simulink model "counter_block"  (R2016b)
settings: Solver=VariableStepAuto  StartTime=0.0  StopTime=10.0  RelTol=1e-3
settings Model: Creator=Lupus  LastModifiedBy=Lupus

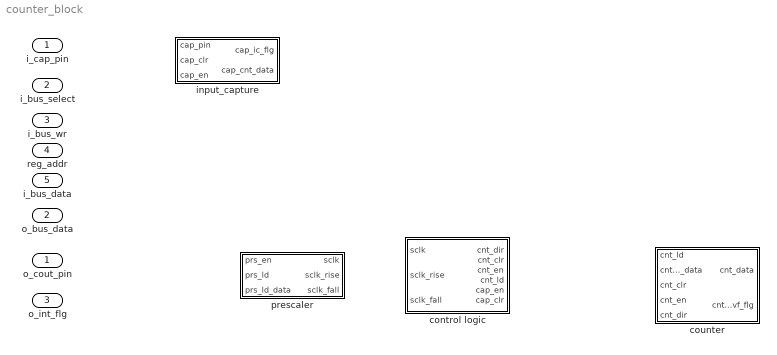
== system counter_block ==
  i_cap_pin : Inport
  i_bus_select : Inport  Port=2
  i_bus_wr : Inport  Port=3
  reg_addr : Inport  Port=4
  i_bus_data : Inport  Port=5
  "control logic " : Subsystem
  counter : Subsystem
  input_capture : Subsystem
  prescaler : Subsystem
  o_cout_pin : Outport
  o_bus_data : Outport  Port=2
  o_int_flg : Outport  Port=3

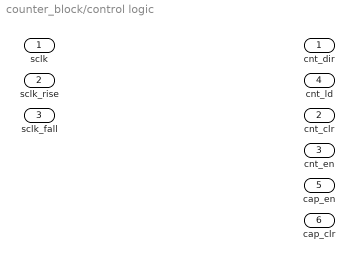
== system counter_block/control logic  ==
  sclk : Inport
  sclk_rise : Inport  Port=2
  sclk_fall : Inport  Port=3
  cnt_dir : Outport
  cnt_clr : Outport  Port=2
  "cnt_en " : Outport  Port=3
  cnt_ld : Outport  Port=4
  cap_en : Outport  Port=5
  cap_clr : Outport  Port=6

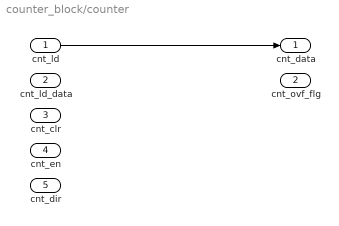
== system counter_block/counter ==
  cnt_ld : Inport
  cnt_ld_data : Inport  Port=2
  cnt_clr : Inport  Port=3
  cnt_en : Inport  Port=4
  cnt_dir : Inport  Port=5
  cnt_data : Outport
  cnt_ovf_flg : Outport  Port=2
  wires:
  cnt_ld/1 -> cnt_data/1

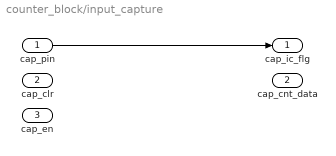
== system counter_block/input_capture ==
  cap_pin : Inport
  cap_clr : Inport  Port=2
  cap_en : Inport  Port=3
  cap_ic_flg : Outport
  cap_cnt_data : Outport  Port=2
  wires:
  cap_pin/1 -> cap_ic_flg/1

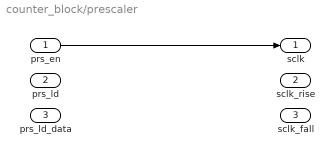
== system counter_block/prescaler ==
  prs_en : Inport
  prs_ld : Inport  Port=2
  prs_ld_data : Inport  Port=3
  sclk : Outport
  sclk_rise : Outport  Port=2
  sclk_fall : Outport  Port=3
  wires:
  prs_en/1 -> sclk/1
